simulink model "test_mdl1"  (R2023a)
settings: Solver=VariableStepAuto  StartTime=0.0  StopTime=10.0  RelTol=1e-3
(part 3 of 8)

== system test_mdl1/VehicleCAN/ECM_Diesel/Stop_Start ==
  AutoStopPtDelta_I_Est : Constant  Value=0
  HiElPwInhbt_B_Stat : Constant  Value=0
  OdoTripVerify_L_Actl : Constant  Value=0
  StopStrtDrvMde_D_Indic : Constant  Value=0
  StopStrtIODTxt_D_Rq : Constant  Value=0
  StopStrtMsgTxt_D_Rq : Constant  Value=0
  StopStrtStdby_D_Indic : Constant  Value=0
  bus_creator : BusCreator  Inputs=7
  out_port : Outport
  wires:
  bus_creator/1 -> out_port/1  "test_mdl1"
  AutoStopPtDelta_I_Est/1 -> bus_creator/1  "AutoStopPtDelta_I_Est"
  HiElPwInhbt_B_Stat/1 -> bus_creator/2  "HiElPwInhbt_B_Stat"
  OdoTripVerify_L_Actl/1 -> bus_creator/3  "OdoTripVerify_L_Actl"
  StopStrtDrvMde_D_Indic/1 -> bus_creator/4  "StopStrtDrvMde_D_Indic"
  StopStrtIODTxt_D_Rq/1 -> bus_creator/5  "StopStrtIODTxt_D_Rq"
  StopStrtMsgTxt_D_Rq/1 -> bus_creator/6  "StopStrtMsgTxt_D_Rq"
  StopStrtStdby_D_Indic/1 -> bus_creator/7  "StopStrtStdby_D_Indic"

== system test_mdl1/VehicleCAN/ECM_Diesel/TesterPhysicalResPCM ==
  TesterPhysicalResPCM : Constant  Value=0
  bus_creator : BusCreator  Inputs=1
  out_port : Outport
  wires:
  bus_creator/1 -> out_port/1  "test_mdl1"
  TesterPhysicalResPCM/1 -> bus_creator/1  "TesterPhysicalResPCM"

== system test_mdl1/VehicleCAN/ECM_Diesel/TesterPhysicalResSOBDMCFD1 ==
  TesterPhysicalResSOBDMC : Constant  Value=0
  bus_creator : BusCreator  Inputs=1
  out_port : Outport
  wires:
  bus_creator/1 -> out_port/1  "test_mdl1"
  TesterPhysicalResSOBDMC/1 -> bus_creator/1  "TesterPhysicalResSOBDMC"

== system test_mdl1/VehicleCAN/ECM_Diesel/TorqueDataEngFlags ==
  PrplWhlTotTqRq_No_Cnt : Constant  Value=0
  PrplWhlTotTqRq_No_Cs : Constant  Value=0
  PrplWhlTot_Tq_LimMn : Constant  Value=0
  PrplWhlTot_Tq_Rq : Constant  Value=0
  PtDrvMde_D_Stat : Constant  Value=0
  bus_creator : BusCreator  Inputs=5
  out_port : Outport
  wires:
  bus_creator/1 -> out_port/1  "test_mdl1"
  PrplWhlTotTqRq_No_Cnt/1 -> bus_creator/1  "PrplWhlTotTqRq_No_Cnt"
  PrplWhlTotTqRq_No_Cs/1 -> bus_creator/2  "PrplWhlTotTqRq_No_Cs"
  PrplWhlTot_Tq_LimMn/1 -> bus_creator/3  "PrplWhlTot_Tq_LimMn"
  PrplWhlTot_Tq_Rq/1 -> bus_creator/4  "PrplWhlTot_Tq_Rq"
  PtDrvMde_D_Stat/1 -> bus_creator/5  "PtDrvMde_D_Stat"

== system test_mdl1/VehicleCAN/ECM_Diesel/VehicleOperatingModes ==
  ElPw_D_Stat : Constant  Value=0
  ElPw_D_StatStrtStop : Constant  Value=0
  Eng_D_Stat : Constant  Value=0
  PlgActvArb_B_Actl : Constant  Value=0
  PrplWhlRgenMn_Tq_Actl : Constant  Value=0
  PrplWhlTot2_Tq_Actl : Constant  Value=0
  PwPckTq_D_Stat : Constant  Value=0
  TrnAinTq_D_Qf : Constant  Value=0
  TrnAin_Tq_Actl : Constant  Value=0
  bus_creator : BusCreator  Inputs=9
  out_port : Outport
  wires:
  bus_creator/1 -> out_port/1  "test_mdl1"
  ElPw_D_Stat/1 -> bus_creator/1  "ElPw_D_Stat"
  ElPw_D_StatStrtStop/1 -> bus_creator/2  "ElPw_D_StatStrtStop"
  Eng_D_Stat/1 -> bus_creator/3  "Eng_D_Stat"
  PlgActvArb_B_Actl/1 -> bus_creator/4  "PlgActvArb_B_Actl"
  PrplWhlRgenMn_Tq_Actl/1 -> bus_creator/5  "PrplWhlRgenMn_Tq_Actl"
  PrplWhlTot2_Tq_Actl/1 -> bus_creator/6  "PrplWhlTot2_Tq_Actl"
  PwPckTq_D_Stat/1 -> bus_creator/7  "PwPckTq_D_Stat"
  TrnAinTq_D_Qf/1 -> bus_creator/8  "TrnAinTq_D_Qf"
  TrnAin_Tq_Actl/1 -> bus_creator/9  "TrnAin_Tq_Actl"

== system test_mdl1/VehicleCAN/GWM/%sonality_APIM_Data_FD1 ==
  %s1OptIn_B_Stats : Constant  Value=0
  %s2OptIn_B_Stats : Constant  Value=0
  %s3OptIn_B_Stats : Constant  Value=0
  %s4OptIn_B_Stats : Constant  Value=0
  %sStore_D_Rq : Constant  Value=0
  CtrStk%sIndex_D_Actl : Constant  Value=0
  CtrStkDsplyOp_D_Rq : Constant  Value=0
  CtrStkFeatConfigActl : Constant  Value=0
  CtrStkFeatNoActl : Constant  Value=0
  bus_creator : BusCreator  Inputs=9
  out_port : Outport
  wires:
  bus_creator/1 -> out_port/1  "test_mdl1"
  CtrStkDsplyOp_D_Rq/1 -> bus_creator/1  "CtrStkDsplyOp_D_Rq"
  CtrStkFeatConfigActl/1 -> bus_creator/2  "CtrStkFeatConfigActl"
  CtrStkFeatNoActl/1 -> bus_creator/3  "CtrStkFeatNoActl"
  CtrStk%sIndex_D_Actl/1 -> bus_creator/4  "CtrStk%sIndex_D_Actl"
  %s1OptIn_B_Stats/1 -> bus_creator/5  "%s1OptIn_B_Stats"
  %s2OptIn_B_Stats/1 -> bus_creator/6  "%s2OptIn_B_Stats"
  %s3OptIn_B_Stats/1 -> bus_creator/7  "%s3OptIn_B_Stats"
  %s4OptIn_B_Stats/1 -> bus_creator/8  "%s4OptIn_B_Stats"
  %sStore_D_Rq/1 -> bus_creator/9  "%sStore_D_Rq"

== system test_mdl1/VehicleCAN/GWM/%sonality_BCM2_Data_FD1 ==
  %s1Key_D_Stat : Constant  Value=0
  %s2Key_D_Stat : Constant  Value=0
  %s3Key_D_Stat : Constant  Value=0
  %s4Key_D_Stat : Constant  Value=0
  %sConflict_D_Actl : Constant  Value=0
  %sNoPos_D_Actl : Constant  Value=0
  %sNo_D_Actl : Constant  Value=0
  %sRecallSrc_D_Actl : Constant  Value=0
  %sSetupAccessCtrl : Constant  Value=0
  %sSetupRestr_D_Actl : Constant  Value=0
  %sSetup_No_Actl : Constant  Value=0
  AssocConfirm_D_Actl : Constant  Value=0
  EmPrflKeyAssoc_D_Stat : Constant  Value=0
  EmPrflNo_D_Stat : Constant  Value=0
  RecallEvent_No_Cnt : Constant  Value=0
  VehKeyActv_D_Stat : Constant  Value=0
  bus_creator : BusCreator  Inputs=16
  out_port : Outport
  wires:
  bus_creator/1 -> out_port/1  "test_mdl1"
  AssocConfirm_D_Actl/1 -> bus_creator/1  "AssocConfirm_D_Actl"
  EmPrflKeyAssoc_D_Stat/1 -> bus_creator/2  "EmPrflKeyAssoc_D_Stat"
  EmPrflNo_D_Stat/1 -> bus_creator/3  "EmPrflNo_D_Stat"
  %s1Key_D_Stat/1 -> bus_creator/4  "%s1Key_D_Stat"
  %s2Key_D_Stat/1 -> bus_creator/5  "%s2Key_D_Stat"
  %s3Key_D_Stat/1 -> bus_creator/6  "%s3Key_D_Stat"
  %s4Key_D_Stat/1 -> bus_creator/7  "%s4Key_D_Stat"
  %sConflict_D_Actl/1 -> bus_creator/8  "%sConflict_D_Actl"
  %sNoPos_D_Actl/1 -> bus_creator/9  "%sNoPos_D_Actl"
  %sNo_D_Actl/1 -> bus_creator/10  "%sNo_D_Actl"
  %sRecallSrc_D_Actl/1 -> bus_creator/11  "%sRecallSrc_D_Actl"
  %sSetupAccessCtrl/1 -> bus_creator/12  "%sSetupAccessCtrl"
  %sSetupRestr_D_Actl/1 -> bus_creator/13  "%sSetupRestr_D_Actl"
  %sSetup_No_Actl/1 -> bus_creator/14  "%sSetup_No_Actl"
  RecallEvent_No_Cnt/1 -> bus_creator/15  "RecallEvent_No_Cnt"
  VehKeyActv_D_Stat/1 -> bus_creator/16  "VehKeyActv_D_Stat"

== system test_mdl1/VehicleCAN/GWM/%sonality_Data_FD1 ==
  MsgCntr%sIndex_D_Rq : Constant  Value=0
  MsgCntrDsplyOp_D_Rq : Constant  Value=0
  MsgCntrFeatConfigRq : Constant  Value=0
  MsgCntrFeatNoRq : Constant  Value=0
  bus_creator : BusCreator  Inputs=4
  out_port : Outport
  wires:
  bus_creator/1 -> out_port/1  "test_mdl1"
  MsgCntrDsplyOp_D_Rq/1 -> bus_creator/1  "MsgCntrDsplyOp_D_Rq"
  MsgCntrFeatConfigRq/1 -> bus_creator/2  "MsgCntrFeatConfigRq"
  MsgCntrFeatNoRq/1 -> bus_creator/3  "MsgCntrFeatNoRq"
  MsgCntr%sIndex_D_Rq/1 -> bus_creator/4  "MsgCntr%sIndex_D_Rq"

== system test_mdl1/VehicleCAN/GWM/AC_Compressor_Data_FD1 ==
  ElCmpr%fErr_D_Falt : Constant  Value=0
  ElCmprBattSysU_D_Falt : Constant  Value=0
  ElCmprBattURng_D_Falt : Constant  Value=0
  ElCmprInnrErr_D_Falt : Constant  Value=0
  ElCmprLostComm_D_Falt : Constant  Value=0
  ElCmprOverLoad_D_Falt : Constant  Value=0
  ElCmprOverTe_D_Falt : Constant  Value=0
  ElCmprOverTe_D_Stat : Constant  Value=0
  ElCmprSysU_D_Falt : Constant  Value=0
  ElCmprUHi_D_Stat : Constant  Value=0
  ElCmprUHi_U_Actl : Constant  Value=0
  ElCmpr_D_Stat : Constant  Value=0
  ElCmpr_N_Actl : Constant  Value=0
  ElCmpr_Pw_Actl : Constant  Value=0
  bus_creator : BusCreator  Inputs=14
  out_port : Outport
  wires:
  bus_creator/1 -> out_port/1  "test_mdl1"
  ElCmprBattSysU_D_Falt/1 -> bus_creator/1  "ElCmprBattSysU_D_Falt"
  ElCmprBattURng_D_Falt/1 -> bus_creator/2  "ElCmprBattURng_D_Falt"
  ElCmprInnrErr_D_Falt/1 -> bus_creator/3  "ElCmprInnrErr_D_Falt"
  ElCmprLostComm_D_Falt/1 -> bus_creator/4  "ElCmprLostComm_D_Falt"
  ElCmprOverLoad_D_Falt/1 -> bus_creator/5  "ElCmprOverLoad_D_Falt"
  ElCmprOverTe_D_Falt/1 -> bus_creator/6  "ElCmprOverTe_D_Falt"
  ElCmprOverTe_D_Stat/1 -> bus_creator/7  "ElCmprOverTe_D_Stat"
  ElCmpr%fErr_D_Falt/1 -> bus_creator/8  "ElCmpr%fErr_D_Falt"
  ElCmprSysU_D_Falt/1 -> bus_creator/9  "ElCmprSysU_D_Falt"
  ElCmprUHi_D_Stat/1 -> bus_creator/10  "ElCmprUHi_D_Stat"
  ElCmprUHi_U_Actl/1 -> bus_creator/11  "ElCmprUHi_U_Actl"
  ElCmpr_D_Stat/1 -> bus_creator/12  "ElCmpr_D_Stat"
  ElCmpr_N_Actl/1 -> bus_creator/13  "ElCmpr_N_Actl"
  ElCmpr_Pw_Actl/1 -> bus_creator/14  "ElCmpr_Pw_Actl"

== system test_mdl1/VehicleCAN/GWM/APIMGPS_Data_Nav_1_FD1 ==
  GPS_Latitude_Degrees : Constant  Value=0
  GPS_Latitude_Min_dec : Constant  Value=0
  GPS_Latitude_Minutes : Constant  Value=0
  GPS_Longitude_Degrees : Constant  Value=0
  GPS_Longitude_Min_dec : Constant  Value=0
  GPS_Longitude_Minutes : Constant  Value=0
  GpsHsphLattSth_D_Actl : Constant  Value=0
  GpsHsphLongEast_D_Actl : Constant  Value=0
  bus_creator : BusCreator  Inputs=8
  out_port : Outport
  wires:
  bus_creator/1 -> out_port/1  "test_mdl1"
  GPS_Latitude_Degrees/1 -> bus_creator/1  "GPS_Latitude_Degrees"
  GPS_Latitude_Min_dec/1 -> bus_creator/2  "GPS_Latitude_Min_dec"
  GPS_Latitude_Minutes/1 -> bus_creator/3  "GPS_Latitude_Minutes"
  GPS_Longitude_Degrees/1 -> bus_creator/4  "GPS_Longitude_Degrees"
  GPS_Longitude_Min_dec/1 -> bus_creator/5  "GPS_Longitude_Min_dec"
  GPS_Longitude_Minutes/1 -> bus_creator/6  "GPS_Longitude_Minutes"
  GpsHsphLattSth_D_Actl/1 -> bus_creator/7  "GpsHsphLattSth_D_Actl"
  GpsHsphLongEast_D_Actl/1 -> bus_creator/8  "GpsHsphLongEast_D_Actl"

== system test_mdl1/VehicleCAN/GWM/APIMGPS_Data_Nav_2_FD1 ==
  GPS_Actual_vs_Infer_pos : Constant  Value=0
  GPS_Compass_direction : Constant  Value=0
  GPS_Pdop : Constant  Value=0
  GPS_UTC_hours : Constant  Value=0
  GPS_UTC_minutes : Constant  Value=0
  GPS_UTC_seconds : Constant  Value=0
  GpsUtcDay_No_Actl : Constant  Value=0
  GpsUtcMnth_No_Actl : Constant  Value=0
  GpsUtcYr_No_Actl : Constant  Value=0
  Gps_B_Falt : Constant  Value=0
  bus_creator : BusCreator  Inputs=10
  out_port : Outport
  wires:
  bus_creator/1 -> out_port/1  "test_mdl1"
  GPS_Actual_vs_Infer_pos/1 -> bus_creator/1  "GPS_Actual_vs_Infer_pos"
  GPS_Compass_direction/1 -> bus_creator/2  "GPS_Compass_direction"
  GPS_Pdop/1 -> bus_creator/3  "GPS_Pdop"
  GPS_UTC_hours/1 -> bus_creator/4  "GPS_UTC_hours"
  GPS_UTC_minutes/1 -> bus_creator/5  "GPS_UTC_minutes"
  GPS_UTC_seconds/1 -> bus_creator/6  "GPS_UTC_seconds"
  GpsUtcDay_No_Actl/1 -> bus_creator/7  "GpsUtcDay_No_Actl"
  GpsUtcMnth_No_Actl/1 -> bus_creator/8  "GpsUtcMnth_No_Actl"
  GpsUtcYr_No_Actl/1 -> bus_creator/9  "GpsUtcYr_No_Actl"
  Gps_B_Falt/1 -> bus_creator/10  "Gps_B_Falt"

== system test_mdl1/VehicleCAN/GWM/APIMGPS_Data_Nav_3_FD1 ==
  GPS_Hdop : Constant  Value=0
  GPS_Heading : Constant  Value=0
  GPS_MSL_altitude : Constant  Value=0
  GPS_Sat_num_in_view : Constant  Value=0
  GPS_Speed : Constant  Value=0
  GPS_Vdop : Constant  Value=0
  GPS_dimension : Constant  Value=0
  bus_creator : BusCreator  Inputs=7
  out_port : Outport
  wires:
  bus_creator/1 -> out_port/1  "test_mdl1"
  GPS_Hdop/1 -> bus_creator/1  "GPS_Hdop"
  GPS_Heading/1 -> bus_creator/2  "GPS_Heading"
  GPS_MSL_altitude/1 -> bus_creator/3  "GPS_MSL_altitude"
  GPS_Sat_num_in_view/1 -> bus_creator/4  "GPS_Sat_num_in_view"
  GPS_Speed/1 -> bus_creator/5  "GPS_Speed"
  GPS_Vdop/1 -> bus_creator/6  "GPS_Vdop"
  GPS_dimension/1 -> bus_creator/7  "GPS_dimension"

== system test_mdl1/VehicleCAN/GWM/APIM_Data_FD1 ==
  AutoLghtOvrrd_B_RqDrv : Constant  Value=0
  DistToStopover_L_Actl : Constant  Value=0
  ExtLghtDsply_D_Stat : Constant  Value=0
  ExtLghtFront_D_RqMnu : Constant  Value=0
  ExtLghtLeft_D_RqMnu : Constant  Value=0
  ExtLghtRear_D_RqMnu : Constant  Value=0
  ExtLghtRight_D_RqMnu : Constant  Value=0
  GoTEditHr_T_RqMnu : Constant  Value=0
  GoTEditMnte_T_RqMnu : Constant  Value=0
  StopoverType_D_Stat : Constant  Value=0
  bus_creator : BusCreator  Inputs=10
  out_port : Outport
  wires:
  bus_creator/1 -> out_port/1  "test_mdl1"
  AutoLghtOvrrd_B_RqDrv/1 -> bus_creator/1  "AutoLghtOvrrd_B_RqDrv"
  DistToStopover_L_Actl/1 -> bus_creator/2  "DistToStopover_L_Actl"
  ExtLghtDsply_D_Stat/1 -> bus_creator/3  "ExtLghtDsply_D_Stat"
  ExtLghtFront_D_RqMnu/1 -> bus_creator/4  "ExtLghtFront_D_RqMnu"
  ExtLghtLeft_D_RqMnu/1 -> bus_creator/5  "ExtLghtLeft_D_RqMnu"
  ExtLghtRear_D_RqMnu/1 -> bus_creator/6  "ExtLghtRear_D_RqMnu"
  ExtLghtRight_D_RqMnu/1 -> bus_creator/7  "ExtLghtRight_D_RqMnu"
  GoTEditHr_T_RqMnu/1 -> bus_creator/8  "GoTEditHr_T_RqMnu"
  GoTEditMnte_T_RqMnu/1 -> bus_creator/9  "GoTEditMnte_T_RqMnu"
  StopoverType_D_Stat/1 -> bus_creator/10  "StopoverType_D_Stat"

== system test_mdl1/VehicleCAN/GWM/APIM_Request_Signals_1_FD1 ==
  Btt_L_Actl2 : Constant  Value=0
  ChrgCrdLckEnbl_B_Stat : Constant  Value=0
  ChrgOvrdExitScrn_D_Rq : Constant  Value=0
  Cntr_Plg_Mode_Cmd : Constant  Value=0
  EmPrflButtnAssoc_D_Rq : Constant  Value=0
  EmPrflKeyAssoc_D_Rq : Constant  Value=0
  EmPrflNo_D_Rq : Constant  Value=0
  Em_D_Stat : Constant  Value=0
  PmCabnLvl_D_Stat : Constant  Value=0
  PmCabn_D_Stat : Constant  Value=0
  PwRnngBoardMde_D_Rq : Constant  Value=0
  PwRnngBoardSwtch_D_Rq : Constant  Value=0
  PwRnngBoardT_D_Rq : Constant  Value=0
  Rba_D_Rq : Constant  Value=0
  bus_creator : BusCreator  Inputs=14
  out_port : Outport
  wires:
  bus_creator/1 -> out_port/1  "test_mdl1"
  Btt_L_Actl2/1 -> bus_creator/1  "Btt_L_Actl2"
  ChrgCrdLckEnbl_B_Stat/1 -> bus_creator/2  "ChrgCrdLckEnbl_B_Stat"
  ChrgOvrdExitScrn_D_Rq/1 -> bus_creator/3  "ChrgOvrdExitScrn_D_Rq"
  Cntr_Plg_Mode_Cmd/1 -> bus_creator/4  "Cntr_Plg_Mode_Cmd"
  EmPrflButtnAssoc_D_Rq/1 -> bus_creator/5  "EmPrflButtnAssoc_D_Rq"
  EmPrflKeyAssoc_D_Rq/1 -> bus_creator/6  "EmPrflKeyAssoc_D_Rq"
  EmPrflNo_D_Rq/1 -> bus_creator/7  "EmPrflNo_D_Rq"
  Em_D_Stat/1 -> bus_creator/8  "Em_D_Stat"
  PmCabnLvl_D_Stat/1 -> bus_creator/9  "PmCabnLvl_D_Stat"
  PmCabn_D_Stat/1 -> bus_creator/10  "PmCabn_D_Stat"
  PwRnngBoardMde_D_Rq/1 -> bus_creator/11  "PwRnngBoardMde_D_Rq"
  PwRnngBoardSwtch_D_Rq/1 -> bus_creator/12  "PwRnngBoardSwtch_D_Rq"
  PwRnngBoardT_D_Rq/1 -> bus_creator/13  "PwRnngBoardT_D_Rq"
  Rba_D_Rq/1 -> bus_creator/14  "Rba_D_Rq"

== system test_mdl1/VehicleCAN/GWM/APIM_Request_Signals_5_FD1 ==
  OnbChrgLocIdTrgt_No_Rq : Constant  Value=0
  OnbChrgLocIdUns_B_Rq : Constant  Value=0
  OnbChrgPrflUpdate_B_Rq : Constant  Value=0
  OnbChrgPrflWkdy_No_Rq : Constant  Value=0
  OnbChrgPrflWknd_No_Rq : Constant  Value=0
  OnbChrgSetDelete_B_Rq : Constant  Value=0
  OnbChrgSetNow_D_Rq : Constant  Value=0
  OnbChrgToPcWkdy_D_Actl : Constant  Value=0
  OnbChrgToPcWknd_D_Actl : Constant  Value=0
  bus_creator : BusCreator  Inputs=9
  out_port : Outport
  wires:
  bus_creator/1 -> out_port/1  "test_mdl1"
  OnbChrgLocIdTrgt_No_Rq/1 -> bus_creator/1  "OnbChrgLocIdTrgt_No_Rq"
  OnbChrgLocIdUns_B_Rq/1 -> bus_creator/2  "OnbChrgLocIdUns_B_Rq"
  OnbChrgPrflUpdate_B_Rq/1 -> bus_creator/3  "OnbChrgPrflUpdate_B_Rq"
  OnbChrgPrflWkdy_No_Rq/1 -> bus_creator/4  "OnbChrgPrflWkdy_No_Rq"
  OnbChrgPrflWknd_No_Rq/1 -> bus_creator/5  "OnbChrgPrflWknd_No_Rq"
  OnbChrgSetDelete_B_Rq/1 -> bus_creator/6  "OnbChrgSetDelete_B_Rq"
  OnbChrgSetNow_D_Rq/1 -> bus_creator/7  "OnbChrgSetNow_D_Rq"
  OnbChrgToPcWkdy_D_Actl/1 -> bus_creator/8  "OnbChrgToPcWkdy_D_Actl"
  OnbChrgToPcWknd_D_Actl/1 -> bus_creator/9  "OnbChrgToPcWknd_D_Actl"

== system test_mdl1/VehicleCAN/GWM/APIM_Request_Signals_FD1 ==
  CbnCmrtPrefListIndx_Rq : Constant  Value=0
  CbnCmrtPrefLstNmItm_Rq : Constant  Value=0
  ChrgStatDsply_D_Rq : Constant  Value=0
  FactoryReset_Rq : Constant  Value=0
  LongTermParking_Rq : Constant  Value=0
  ModemReset_D_Rq : Constant  Value=0
  NextUsageTimeToggle_Rq : Constant  Value=0
  OffPeakTimeSetHR_Rq : Constant  Value=0
  OffPeakTimeSetMin_Rq : Constant  Value=0
  StopStrtDrvMde_B_RqBtn3 : Constant  Value=0
  TCU_ESN_D_Rq : Constant  Value=0
  bus_creator : BusCreator  Inputs=11
  out_port : Outport
  wires:
  bus_creator/1 -> out_port/1  "test_mdl1"
  CbnCmrtPrefListIndx_Rq/1 -> bus_creator/1  "CbnCmrtPrefListIndx_Rq"
  CbnCmrtPrefLstNmItm_Rq/1 -> bus_creator/2  "CbnCmrtPrefLstNmItm_Rq"
  ChrgStatDsply_D_Rq/1 -> bus_creator/3  "ChrgStatDsply_D_Rq"
  FactoryReset_Rq/1 -> bus_creator/4  "FactoryReset_Rq"
  LongTermParking_Rq/1 -> bus_creator/5  "LongTermParking_Rq"
  ModemReset_D_Rq/1 -> bus_creator/6  "ModemReset_D_Rq"
  NextUsageTimeToggle_Rq/1 -> bus_creator/7  "NextUsageTimeToggle_Rq"
  OffPeakTimeSetHR_Rq/1 -> bus_creator/8  "OffPeakTimeSetHR_Rq"
  OffPeakTimeSetMin_Rq/1 -> bus_creator/9  "OffPeakTimeSetMin_Rq"
  StopStrtDrvMde_B_RqBtn3/1 -> bus_creator/10  "StopStrtDrvMde_B_RqBtn3"
  TCU_ESN_D_Rq/1 -> bus_creator/11  "TCU_ESN_D_Rq"

== system test_mdl1/VehicleCAN/GWM/APIM_Send_Signals1_FD1 ==
  APIM_ActiveTrackNum_St : Constant  Value=0
  APIM_NumberofTracks_St : Constant  Value=0
  AutoHoldSwtch_D_Stat3 : Constant  Value=0
  CenterStackRing_D_Actl : Constant  Value=0
  ChrgCordUnlock_B_Rq : Constant  Value=0
  TrlrAidCancl_B_Rq : Constant  Value=0
  TrlrAidSetup_D_Stat : Constant  Value=0
  TrlrTrgtAcquire_D_Rq : Constant  Value=0
  ValetMode_D_Stat : Constant  Value=0
  bus_creator : BusCreator  Inputs=9
  out_port : Outport
  wires:
  bus_creator/1 -> out_port/1  "test_mdl1"
  APIM_ActiveTrackNum_St/1 -> bus_creator/1  "APIM_ActiveTrackNum_St"
  APIM_NumberofTracks_St/1 -> bus_creator/2  "APIM_NumberofTracks_St"
  AutoHoldSwtch_D_Stat3/1 -> bus_creator/3  "AutoHoldSwtch_D_Stat3"
  CenterStackRing_D_Actl/1 -> bus_creator/4  "CenterStackRing_D_Actl"
  ChrgCordUnlock_B_Rq/1 -> bus_creator/5  "ChrgCordUnlock_B_Rq"
  TrlrAidCancl_B_Rq/1 -> bus_creator/6  "TrlrAidCancl_B_Rq"
  TrlrAidSetup_D_Stat/1 -> bus_creator/7  "TrlrAidSetup_D_Stat"
  TrlrTrgtAcquire_D_Rq/1 -> bus_creator/8  "TrlrTrgtAcquire_D_Rq"
  ValetMode_D_Stat/1 -> bus_creator/9  "ValetMode_D_Stat"

== system test_mdl1/VehicleCAN/GWM/APIM_Send_Signals_2_FD1 ==
  AutoEpbButtn_B_Stat : Constant  Value=0
  AutoEpbZoomView_B_Stat : Constant  Value=0
  DcacGfciTestBttn_B_Stat : Constant  Value=0
  DcacPwButtn_B_Falt : Constant  Value=0
  DcacPwHiButtn_B_Stat : Constant  Value=0
  DcacPwLoButtn_B_Stat : Constant  Value=0
  DcacPwOffButtn_B_Stat : Constant  Value=0
  DcacPwResetButtn_B_Stat : Constant  Value=0
  OnbChrgClearAll_B_Rq : Constant  Value=0
  OnbChrgGoTDelete_B_Rq : Constant  Value=0
  OnbChrgGoTElement_D_Rq : Constant  Value=0
  OnbChrgGoTExtHtr_D_Rq : Constant  Value=0
  OnbChrgGoTHr_T_Rq : Constant  Value=0
  OnbChrgGoTMnte_D_Rq : Constant  Value=0
  OnbChrgGoTOn_D_Rq : Constant  Value=0
  OnbChrgGoTPrcond_D_Rq : Constant  Value=0
  OnbChrgGoTTouch_D_Rq : Constant  Value=0
  OnbChrgGoTUpdate_B_Rq : Constant  Value=0
  OtaTrg_D_Stat : Constant  Value=0
  PaakMyKey_D_Rq : Constant  Value=0
  TCU_Final_Actvtn_St : Constant  Value=0
  TCU_Init_Actvtn_St : Constant  Value=0
  TrlrAidMde_D_Rq : Constant  Value=0
  TrlrBrkGain_No_Rq : Constant  Value=0
  TrlrHitch_D_RqMnu : Constant  Value=0
  bus_creator : BusCreator  Inputs=25
  out_port : Outport
  wires:
  bus_creator/1 -> out_port/1  "test_mdl1"
  AutoEpbButtn_B_Stat/1 -> bus_creator/1  "AutoEpbButtn_B_Stat"
  AutoEpbZoomView_B_Stat/1 -> bus_creator/2  "AutoEpbZoomView_B_Stat"
  DcacGfciTestBttn_B_Stat/1 -> bus_creator/3  "DcacGfciTestBttn_B_Stat"
  DcacPwButtn_B_Falt/1 -> bus_creator/4  "DcacPwButtn_B_Falt"
  DcacPwHiButtn_B_Stat/1 -> bus_creator/5  "DcacPwHiButtn_B_Stat"
  DcacPwLoButtn_B_Stat/1 -> bus_creator/6  "DcacPwLoButtn_B_Stat"
  DcacPwOffButtn_B_Stat/1 -> bus_creator/7  "DcacPwOffButtn_B_Stat"
  DcacPwResetButtn_B_Stat/1 -> bus_creator/8  "DcacPwResetButtn_B_Stat"
  OnbChrgClearAll_B_Rq/1 -> bus_creator/9  "OnbChrgClearAll_B_Rq"
  OnbChrgGoTDelete_B_Rq/1 -> bus_creator/10  "OnbChrgGoTDelete_B_Rq"
  OnbChrgGoTElement_D_Rq/1 -> bus_creator/11  "OnbChrgGoTElement_D_Rq"
  OnbChrgGoTExtHtr_D_Rq/1 -> bus_creator/12  "OnbChrgGoTExtHtr_D_Rq"
  OnbChrgGoTHr_T_Rq/1 -> bus_creator/13  "OnbChrgGoTHr_T_Rq"
  OnbChrgGoTMnte_D_Rq/1 -> bus_creator/14  "OnbChrgGoTMnte_D_Rq"
  OnbChrgGoTOn_D_Rq/1 -> bus_creator/15  "OnbChrgGoTOn_D_Rq"
  OnbChrgGoTPrcond_D_Rq/1 -> bus_creator/16  "OnbChrgGoTPrcond_D_Rq"
  OnbChrgGoTTouch_D_Rq/1 -> bus_creator/17  "OnbChrgGoTTouch_D_Rq"
  OnbChrgGoTUpdate_B_Rq/1 -> bus_creator/18  "OnbChrgGoTUpdate_B_Rq"
  OtaTrg_D_Stat/1 -> bus_creator/19  "OtaTrg_D_Stat"
  PaakMyKey_D_Rq/1 -> bus_creator/20  "PaakMyKey_D_Rq"
  TCU_Final_Actvtn_St/1 -> bus_creator/21  "TCU_Final_Actvtn_St"
  TCU_Init_Actvtn_St/1 -> bus_creator/22  "TCU_Init_Actvtn_St"
  TrlrAidMde_D_Rq/1 -> bus_creator/23  "TrlrAidMde_D_Rq"
  TrlrBrkGain_No_Rq/1 -> bus_creator/24  "TrlrBrkGain_No_Rq"
  TrlrHitch_D_RqMnu/1 -> bus_creator/25  "TrlrHitch_D_RqMnu"

== system test_mdl1/VehicleCAN/GWM/Accel_Data_FD1 ==
  VehLat2_A_Actl : Constant  Value=0
  VehLatAActl_D_Qf : Constant  Value=0
  VehLatLongVertA_No_Cs : Constant  Value=0
  VehLatLongVert_No_Cnt : Constant  Value=0
  VehLong2_A_Actl : Constant  Value=0
  VehLongAActl_D_Qf : Constant  Value=0
  VehVert2_A_Actl : Constant  Value=0
  VehVertAActl_D_Qf : Constant  Value=0
  bus_creator : BusCreator  Inputs=8
  out_port : Outport
  wires:
  bus_creator/1 -> out_port/1  "test_mdl1"
  VehLat2_A_Actl/1 -> bus_creator/1  "VehLat2_A_Actl"
  VehLatAActl_D_Qf/1 -> bus_creator/2  "VehLatAActl_D_Qf"
  VehLatLongVertA_No_Cs/1 -> bus_creator/3  "VehLatLongVertA_No_Cs"
  VehLatLongVert_No_Cnt/1 -> bus_creator/4  "VehLatLongVert_No_Cnt"
  VehLong2_A_Actl/1 -> bus_creator/5  "VehLong2_A_Actl"
  VehLongAActl_D_Qf/1 -> bus_creator/6  "VehLongAActl_D_Qf"
  VehVert2_A_Actl/1 -> bus_creator/7  "VehVert2_A_Actl"
  VehVertAActl_D_Qf/1 -> bus_creator/8  "VehVertAActl_D_Qf"

== system test_mdl1/VehicleCAN/GWM/ActiveFrontStrg_Stat2_FD1 ==
  SteWhlRelCalib_An_Sns : Constant  Value=0
  SteWhlRelCalib_T_Actl : Constant  Value=0
  bus_creator : BusCreator  Inputs=2
  out_port : Outport
  wires:
  bus_creator/1 -> out_port/1  "test_mdl1"
  SteWhlRelCalib_An_Sns/1 -> bus_creator/1  "SteWhlRelCalib_An_Sns"
  SteWhlRelCalib_T_Actl/1 -> bus_creator/2  "SteWhlRelCalib_T_Actl"

== system test_mdl1/VehicleCAN/GWM/ActiveFrontStrg_Stat_FD1 ==
  SteWhlBrkAnActl_No_Cnt : Constant  Value=0
  SteWhlBrkAnActl_No_Cs : Constant  Value=0
  SteWhlBrkOffst_An_Actl : Constant  Value=0
  SteWhlOffstRq_D_Stat : Constant  Value=0
  SteWhlOffst_An_TotActl : Constant  Value=0
  bus_creator : BusCreator  Inputs=5
  out_port : Outport
  wires:
  bus_creator/1 -> out_port/1  "test_mdl1"
  SteWhlBrkAnActl_No_Cnt/1 -> bus_creator/1  "SteWhlBrkAnActl_No_Cnt"
  SteWhlBrkAnActl_No_Cs/1 -> bus_creator/2  "SteWhlBrkAnActl_No_Cs"
  SteWhlBrkOffst_An_Actl/1 -> bus_creator/3  "SteWhlBrkOffst_An_Actl"
  SteWhlOffstRq_D_Stat/1 -> bus_creator/4  "SteWhlOffstRq_D_Stat"
  SteWhlOffst_An_TotActl/1 -> bus_creator/5  "SteWhlOffst_An_TotActl"

== system test_mdl1/VehicleCAN/GWM/Adaptive_Headlamp_Stat ==
  Adaptive_Hdlmp_Fault : Constant  Value=0
  AhbStatGfhbFdbk_D_Actl : Constant  Value=0
  HeadLghtDrvSide_B_Stat : Constant  Value=0
  HeadLghtHiOn_B_StatHcm : Constant  Value=0
  bus_creator : BusCreator  Inputs=4
  out_port : Outport
  wires:
  bus_creator/1 -> out_port/1  "test_mdl1"
  Adaptive_Hdlmp_Fault/1 -> bus_creator/1  "Adaptive_Hdlmp_Fault"
  AhbStatGfhbFdbk_D_Actl/1 -> bus_creator/2  "AhbStatGfhbFdbk_D_Actl"
  HeadLghtDrvSide_B_Stat/1 -> bus_creator/3  "HeadLghtDrvSide_B_Stat"
  HeadLghtHiOn_B_StatHcm/1 -> bus_creator/4  "HeadLghtHiOn_B_StatHcm"

== system test_mdl1/VehicleCAN/GWM/AllTerrainControlData_FD1 ==
  SelDrvMdeCnt_D_Stat : Constant  Value=0
  SelDrvMdeSwtch_D_Stat : Constant  Value=0
  SelDrvMdeSwtch_No_Actl : Constant  Value=0
  bus_creator : BusCreator  Inputs=3
  out_port : Outport
  wires:
  bus_creator/1 -> out_port/1  "test_mdl1"
  SelDrvMdeCnt_D_Stat/1 -> bus_creator/1  "SelDrvMdeCnt_D_Stat"
  SelDrvMdeSwtch_D_Stat/1 -> bus_creator/2  "SelDrvMdeSwtch_D_Stat"
  SelDrvMdeSwtch_No_Actl/1 -> bus_creator/3  "SelDrvMdeSwtch_No_Actl"

== system test_mdl1/VehicleCAN/GWM/All_Terrain_Data_FD1 ==
  TerrMde_D_RqDrv : Constant  Value=0
  bus_creator : BusCreator  Inputs=1
  out_port : Outport
  wires:
  bus_creator/1 -> out_port/1  "test_mdl1"
  TerrMde_D_RqDrv/1 -> bus_creator/1  "TerrMde_D_RqDrv"

== system test_mdl1/VehicleCAN/GWM/BCMC_Data_FD1 ==
  WndwRearHeat_D_Stat : Constant  Value=0
  WndwRearHeat_I_Actl : Constant  Value=0
  bus_creator : BusCreator  Inputs=2
  out_port : Outport
  wires:
  bus_creator/1 -> out_port/1  "test_mdl1"
  WndwRearHeat_D_Stat/1 -> bus_creator/1  "WndwRearHeat_D_Stat"
  WndwRearHeat_I_Actl/1 -> bus_creator/2  "WndwRearHeat_I_Actl"

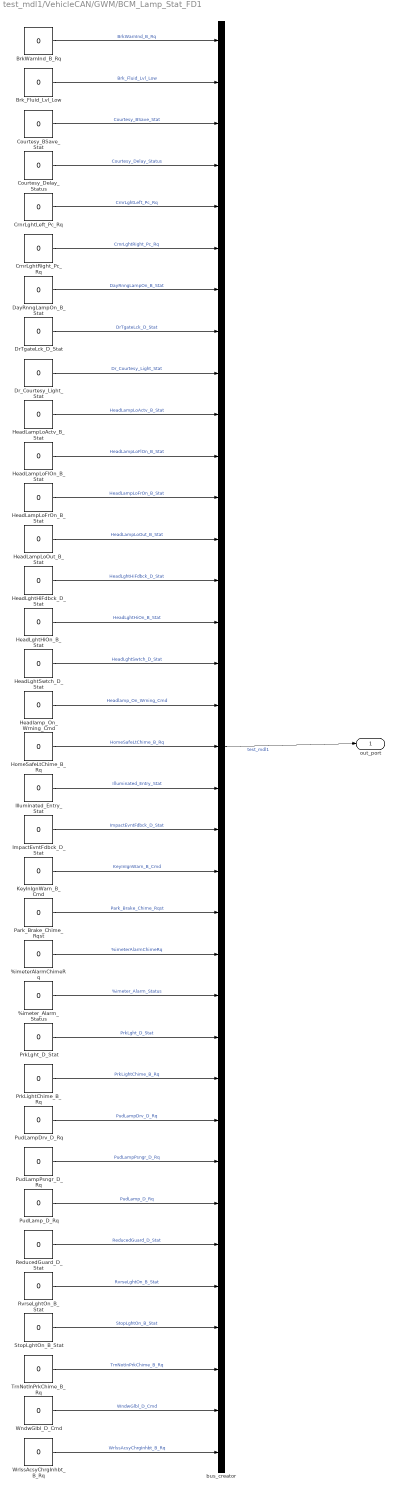
== system test_mdl1/VehicleCAN/GWM/BCM_Lamp_Stat_FD1 ==
  %imeterAlarmChimeRq : Constant  Value=0
  %imeter_Alarm_Status : Constant  Value=0
  BrkWarnInd_B_Rq : Constant  Value=0
  Brk_Fluid_Lvl_Low : Constant  Value=0
  Courtesy_BSave_Stat : Constant  Value=0
  Courtesy_Delay_Status : Constant  Value=0
  CrnrLghtLeft_Pc_Rq : Constant  Value=0
  CrnrLghtRight_Pc_Rq : Constant  Value=0
  DayRnngLampOn_B_Stat : Constant  Value=0
  DrTgateLck_D_Stat : Constant  Value=0
  Dr_Courtesy_Light_Stat : Constant  Value=0
  HeadLampLoActv_B_Stat : Constant  Value=0
  HeadLampLoFlOn_B_Stat : Constant  Value=0
  HeadLampLoFrOn_B_Stat : Constant  Value=0
  HeadLampLoOut_B_Stat : Constant  Value=0
  HeadLghtHiFdbck_D_Stat : Constant  Value=0
  HeadLghtHiOn_B_Stat : Constant  Value=0
  HeadLghtSwtch_D_Stat : Constant  Value=0
  Headlamp_On_Wrning_Cmd : Constant  Value=0
  HomeSafeLtChime_B_Rq : Constant  Value=0
  Illuminated_Entry_Stat : Constant  Value=0
  ImpactEvntFdbck_D_Stat : Constant  Value=0
  KeyInIgnWarn_B_Cmd : Constant  Value=0
  Park_Brake_Chime_Rqst : Constant  Value=0
  PrkLght_D_Stat : Constant  Value=0
  PrkLightChime_B_Rq : Constant  Value=0
  PudLampDrv_D_Rq : Constant  Value=0
  PudLampPsngr_D_Rq : Constant  Value=0
  PudLamp_D_Rq : Constant  Value=0
  ReducedGuard_D_Stat : Constant  Value=0
  RvrseLghtOn_B_Stat : Constant  Value=0
  StopLghtOn_B_Stat : Constant  Value=0
  TrnNotInPrkChime_B_Rq : Constant  Value=0
  WndwGlbl_D_Cmd : Constant  Value=0
  WrlssAcsyChrgInhbt_B_Rq : Constant  Value=0
  bus_creator : BusCreator  Inputs=35
  out_port : Outport
  wires:
  bus_creator/1 -> out_port/1  "test_mdl1"
  BrkWarnInd_B_Rq/1 -> bus_creator/1  "BrkWarnInd_B_Rq"
  Brk_Fluid_Lvl_Low/1 -> bus_creator/2  "Brk_Fluid_Lvl_Low"
  Courtesy_BSave_Stat/1 -> bus_creator/3  "Courtesy_BSave_Stat"
  Courtesy_Delay_Status/1 -> bus_creator/4  "Courtesy_Delay_Status"
  CrnrLghtLeft_Pc_Rq/1 -> bus_creator/5  "CrnrLghtLeft_Pc_Rq"
  CrnrLghtRight_Pc_Rq/1 -> bus_creator/6  "CrnrLghtRight_Pc_Rq"
  DayRnngLampOn_B_Stat/1 -> bus_creator/7  "DayRnngLampOn_B_Stat"
  DrTgateLck_D_Stat/1 -> bus_creator/8  "DrTgateLck_D_Stat"
  Dr_Courtesy_Light_Stat/1 -> bus_creator/9  "Dr_Courtesy_Light_Stat"
  HeadLampLoActv_B_Stat/1 -> bus_creator/10  "HeadLampLoActv_B_Stat"
  HeadLampLoFlOn_B_Stat/1 -> bus_creator/11  "HeadLampLoFlOn_B_Stat"
  HeadLampLoFrOn_B_Stat/1 -> bus_creator/12  "HeadLampLoFrOn_B_Stat"
  HeadLampLoOut_B_Stat/1 -> bus_creator/13  "HeadLampLoOut_B_Stat"
  HeadLghtHiFdbck_D_Stat/1 -> bus_creator/14  "HeadLghtHiFdbck_D_Stat"
  HeadLghtHiOn_B_Stat/1 -> bus_creator/15  "HeadLghtHiOn_B_Stat"
  HeadLghtSwtch_D_Stat/1 -> bus_creator/16  "HeadLghtSwtch_D_Stat"
  Headlamp_On_Wrning_Cmd/1 -> bus_creator/17  "Headlamp_On_Wrning_Cmd"
  HomeSafeLtChime_B_Rq/1 -> bus_creator/18  "HomeSafeLtChime_B_Rq"
  Illuminated_Entry_Stat/1 -> bus_creator/19  "Illuminated_Entry_Stat"
  ImpactEvntFdbck_D_Stat/1 -> bus_creator/20  "ImpactEvntFdbck_D_Stat"
  KeyInIgnWarn_B_Cmd/1 -> bus_creator/21  "KeyInIgnWarn_B_Cmd"
  Park_Brake_Chime_Rqst/1 -> bus_creator/22  "Park_Brake_Chime_Rqst"
  %imeterAlarmChimeRq/1 -> bus_creator/23  "%imeterAlarmChimeRq"
  %imeter_Alarm_Status/1 -> bus_creator/24  "%imeter_Alarm_Status"
  PrkLght_D_Stat/1 -> bus_creator/25  "PrkLght_D_Stat"
  PrkLightChime_B_Rq/1 -> bus_creator/26  "PrkLightChime_B_Rq"
  PudLampDrv_D_Rq/1 -> bus_creator/27  "PudLampDrv_D_Rq"
  PudLampPsngr_D_Rq/1 -> bus_creator/28  "PudLampPsngr_D_Rq"
  PudLamp_D_Rq/1 -> bus_creator/29  "PudLamp_D_Rq"
  ReducedGuard_D_Stat/1 -> bus_creator/30  "ReducedGuard_D_Stat"
  RvrseLghtOn_B_Stat/1 -> bus_creator/31  "RvrseLghtOn_B_Stat"
  StopLghtOn_B_Stat/1 -> bus_creator/32  "StopLghtOn_B_Stat"
  TrnNotInPrkChime_B_Rq/1 -> bus_creator/33  "TrnNotInPrkChime_B_Rq"
  WndwGlbl_D_Cmd/1 -> bus_creator/34  "WndwGlbl_D_Cmd"
  WrlssAcsyChrgInhbt_B_Rq/1 -> bus_creator/35  "WrlssAcsyChrgInhbt_B_Rq"

== system test_mdl1/VehicleCAN/GWM/BattRgenLo_1_FD1 ==
  BattRgenLo_I_Actl : Constant  Value=0
  BattRgenLo_U_Actl : Constant  Value=0
  bus_creator : BusCreator  Inputs=2
  out_port : Outport
  wires:
  bus_creator/1 -> out_port/1  "test_mdl1"
  BattRgenLo_I_Actl/1 -> bus_creator/1  "BattRgenLo_I_Actl"
  BattRgenLo_U_Actl/1 -> bus_creator/2  "BattRgenLo_U_Actl"

== system test_mdl1/VehicleCAN/GWM/BattRgenLo_2_FD1 ==
  BattRgenLoChrg_I_Mx : Constant  Value=0
  BattRgenLoChrg_U_Mx : Constant  Value=0
  BattRgenLoDchrg_I_Mx : Constant  Value=0
  BattRgenLoDchrg_U_Mn : Constant  Value=0
  BattRgenLoOpen_U_Actl : Constant  Value=0
  bus_creator : BusCreator  Inputs=5
  out_port : Outport
  wires:
  bus_creator/1 -> out_port/1  "test_mdl1"
  BattRgenLoChrg_I_Mx/1 -> bus_creator/1  "BattRgenLoChrg_I_Mx"
  BattRgenLoChrg_U_Mx/1 -> bus_creator/2  "BattRgenLoChrg_U_Mx"
  BattRgenLoDchrg_I_Mx/1 -> bus_creator/3  "BattRgenLoDchrg_I_Mx"
  BattRgenLoDchrg_U_Mn/1 -> bus_creator/4  "BattRgenLoDchrg_U_Mn"
  BattRgenLoOpen_U_Actl/1 -> bus_creator/5  "BattRgenLoOpen_U_Actl"

== system test_mdl1/VehicleCAN/GWM/BattRgenLo_3_FD1 ==
  BattRgenLoBalnc_B_Rq : Constant  Value=0
  BattRgenLo_AhRide_Actl : Constant  Value=0
  BattRgenLo_Ah_Actl : Constant  Value=0
  BattRgenLo_R_Actl : Constant  Value=0
  BattRgenLo_Te_Actl : Constant  Value=0
  BattRgenLo_Te_Hi : Constant  Value=0
  bus_creator : BusCreator  Inputs=6
  out_port : Outport
  wires:
  bus_creator/1 -> out_port/1  "test_mdl1"
  BattRgenLoBalnc_B_Rq/1 -> bus_creator/1  "BattRgenLoBalnc_B_Rq"
  BattRgenLo_AhRide_Actl/1 -> bus_creator/2  "BattRgenLo_AhRide_Actl"
  BattRgenLo_Ah_Actl/1 -> bus_creator/3  "BattRgenLo_Ah_Actl"
  BattRgenLo_R_Actl/1 -> bus_creator/4  "BattRgenLo_R_Actl"
  BattRgenLo_Te_Actl/1 -> bus_creator/5  "BattRgenLo_Te_Actl"
  BattRgenLo_Te_Hi/1 -> bus_creator/6  "BattRgenLo_Te_Hi"

== system test_mdl1/VehicleCAN/GWM/BattRgenLo_4_FD1 ==
  BattRgenLoChrg_B_Rq : Constant  Value=0
  BattRgenLoChrg_D_Stat : Constant  Value=0
  BattRgenLoDChrg_D_Stat : Constant  Value=0
  BattRgenLoDchrg_B_Rq : Constant  Value=0
  BattRgenLoPrtct_B_Stat : Constant  Value=0
  BattRgenLoPulse_U_Pred : Constant  Value=0
  BattRgenLoSoc_Pc_Actl : Constant  Value=0
  BattRgenLoStat_D_Qlty : Constant  Value=0
  BattRgenLo_B_Falt : Constant  Value=0
  BattRgenLo_T_Est : Constant  Value=0
  bus_creator : BusCreator  Inputs=10
  out_port : Outport
  wires:
  bus_creator/1 -> out_port/1  "test_mdl1"
  BattRgenLoChrg_B_Rq/1 -> bus_creator/1  "BattRgenLoChrg_B_Rq"
  BattRgenLoChrg_D_Stat/1 -> bus_creator/2  "BattRgenLoChrg_D_Stat"
  BattRgenLoDChrg_D_Stat/1 -> bus_creator/3  "BattRgenLoDChrg_D_Stat"
  BattRgenLoDchrg_B_Rq/1 -> bus_creator/4  "BattRgenLoDchrg_B_Rq"
  BattRgenLoPrtct_B_Stat/1 -> bus_creator/5  "BattRgenLoPrtct_B_Stat"
  BattRgenLoPulse_U_Pred/1 -> bus_creator/6  "BattRgenLoPulse_U_Pred"
  BattRgenLoSoc_Pc_Actl/1 -> bus_creator/7  "BattRgenLoSoc_Pc_Actl"
  BattRgenLoStat_D_Qlty/1 -> bus_creator/8  "BattRgenLoStat_D_Qlty"
  BattRgenLo_B_Falt/1 -> bus_creator/9  "BattRgenLo_B_Falt"
  BattRgenLo_T_Est/1 -> bus_creator/10  "BattRgenLo_T_Est"

== system test_mdl1/VehicleCAN/GWM/Battery_Mgmt_24V_FD1 ==
  BattULo24Soc_Pc_Actl : Constant  Value=0
  BattULo24State_D_Qlty : Constant  Value=0
  BattULo24_Ah_DeltaRide : Constant  Value=0
  BattULo24_B_Falt : Constant  Value=0
  BattULo24_D_Falt : Constant  Value=0
  BattULo24_I_Actl : Constant  Value=0
  BattULo24_Te_Actl : Constant  Value=0
  bus_creator : BusCreator  Inputs=7
  out_port : Outport
  wires:
  bus_creator/1 -> out_port/1  "test_mdl1"
  BattULo24Soc_Pc_Actl/1 -> bus_creator/1  "BattULo24Soc_Pc_Actl"
  BattULo24State_D_Qlty/1 -> bus_creator/2  "BattULo24State_D_Qlty"
  BattULo24_Ah_DeltaRide/1 -> bus_creator/3  "BattULo24_Ah_DeltaRide"
  BattULo24_B_Falt/1 -> bus_creator/4  "BattULo24_B_Falt"
  BattULo24_D_Falt/1 -> bus_creator/5  "BattULo24_D_Falt"
  BattULo24_I_Actl/1 -> bus_creator/6  "BattULo24_I_Actl"
  BattULo24_Te_Actl/1 -> bus_creator/7  "BattULo24_Te_Actl"

== system test_mdl1/VehicleCAN/GWM/Battery_Mgmt_2_FD1 ==
  %iodicElLoad_B_Stat : Constant  Value=0
  BattULoChrg_D_Rq : Constant  Value=0
  BattULoSrvc_T_Actl : Constant  Value=0
  Batt_Crit_SoC_B : Constant  Value=0
  Batt_Lo_SoC_B : Constant  Value=0
  ChargeMode : Constant  Value=0
  EngStrtInhbt_B_RqBatt : Constant  Value=0
  IdleSpeedIncrease_El : Constant  Value=0
  PwSysULoFalt_D_Stat : Constant  Value=0
  Shed_Drain_Eng_Off_B : Constant  Value=0
  Shed_Feature_Group_ID : Constant  Value=0
  Shed_Level_Req : Constant  Value=0
  Shed_T_Eng_Off_B : Constant  Value=0
  ULoRgenTestMde_B_Rq : Constant  Value=0
  bus_creator : BusCreator  Inputs=14
  out_port : Outport
  wires:
  bus_creator/1 -> out_port/1  "test_mdl1"
  BattULoChrg_D_Rq/1 -> bus_creator/1  "BattULoChrg_D_Rq"
  BattULoSrvc_T_Actl/1 -> bus_creator/2  "BattULoSrvc_T_Actl"
  Batt_Crit_SoC_B/1 -> bus_creator/3  "Batt_Crit_SoC_B"
  Batt_Lo_SoC_B/1 -> bus_creator/4  "Batt_Lo_SoC_B"
  ChargeMode/1 -> bus_creator/5  "ChargeMode"
  EngStrtInhbt_B_RqBatt/1 -> bus_creator/6  "EngStrtInhbt_B_RqBatt"
  IdleSpeedIncrease_El/1 -> bus_creator/7  "IdleSpeedIncrease_El"
  %iodicElLoad_B_Stat/1 -> bus_creator/8  "%iodicElLoad_B_Stat"
  PwSysULoFalt_D_Stat/1 -> bus_creator/9  "PwSysULoFalt_D_Stat"
  Shed_Drain_Eng_Off_B/1 -> bus_creator/10  "Shed_Drain_Eng_Off_B"
  Shed_Feature_Group_ID/1 -> bus_creator/11  "Shed_Feature_Group_ID"
  Shed_Level_Req/1 -> bus_creator/12  "Shed_Level_Req"
  Shed_T_Eng_Off_B/1 -> bus_creator/13  "Shed_T_Eng_Off_B"
  ULoRgenTestMde_B_Rq/1 -> bus_creator/14  "ULoRgenTestMde_B_Rq"

== system test_mdl1/VehicleCAN/GWM/Battery_Mgmt_3_FD1 ==
  BSBattQCapAh : Constant  Value=0
  BSBattQDeltaRideAh : Constant  Value=0
  BSBattSOC : Constant  Value=0
  BSFault : Constant  Value=0
  BattULo2_Te_Actl : Constant  Value=0
  BattULoChrg_URate_RqMx : Constant  Value=0
  BattULoChrg_U_RqMn : Constant  Value=0
  BattULoChrg_U_RqMx : Constant  Value=0
  BattULoState_D_Qlty : Constant  Value=0
  bus_creator : BusCreator  Inputs=9
  out_port : Outport
  wires:
  bus_creator/1 -> out_port/1  "test_mdl1"
  BSBattQCapAh/1 -> bus_creator/1  "BSBattQCapAh"
  BSBattQDeltaRideAh/1 -> bus_creator/2  "BSBattQDeltaRideAh"
  BSBattSOC/1 -> bus_creator/3  "BSBattSOC"
  BSFault/1 -> bus_creator/4  "BSFault"
  BattULo2_Te_Actl/1 -> bus_creator/5  "BattULo2_Te_Actl"
  BattULoChrg_URate_RqMx/1 -> bus_creator/6  "BattULoChrg_URate_RqMx"
  BattULoChrg_U_RqMn/1 -> bus_creator/7  "BattULoChrg_U_RqMn"
  BattULoChrg_U_RqMx/1 -> bus_creator/8  "BattULoChrg_U_RqMx"
  BattULoState_D_Qlty/1 -> bus_creator/9  "BattULoState_D_Qlty"

== system test_mdl1/VehicleCAN/GWM/Battery_Mgmt_4_FD1 ==
  BattULoAuxIsol_D_Rq : Constant  Value=0
  BattULoAuxSoc_Pc_Actl : Constant  Value=0
  BattULoAux_B_Falt : Constant  Value=0
  BattULoAux_D_Qlty : Constant  Value=0
  BattULoAux_I_Actl : Constant  Value=0
  BattULoAux_U_Actl : Constant  Value=0
  BattULoAux_U_Rq : Constant  Value=0
  BattULoCrnkBelt_U_Pred : Constant  Value=0
  BattULoCrnkStrt_U_Pred : Constant  Value=0
  bus_creator : BusCreator  Inputs=9
  out_port : Outport
  wires:
  bus_creator/1 -> out_port/1  "test_mdl1"
  BattULoAuxIsol_D_Rq/1 -> bus_creator/1  "BattULoAuxIsol_D_Rq"
  BattULoAuxSoc_Pc_Actl/1 -> bus_creator/2  "BattULoAuxSoc_Pc_Actl"
  BattULoAux_B_Falt/1 -> bus_creator/3  "BattULoAux_B_Falt"
  BattULoAux_D_Qlty/1 -> bus_creator/4  "BattULoAux_D_Qlty"
  BattULoAux_I_Actl/1 -> bus_creator/5  "BattULoAux_I_Actl"
  BattULoAux_U_Actl/1 -> bus_creator/6  "BattULoAux_U_Actl"
  BattULoAux_U_Rq/1 -> bus_creator/7  "BattULoAux_U_Rq"
  BattULoCrnkBelt_U_Pred/1 -> bus_creator/8  "BattULoCrnkBelt_U_Pred"
  BattULoCrnkStrt_U_Pred/1 -> bus_creator/9  "BattULoCrnkStrt_U_Pred"

== system test_mdl1/VehicleCAN/GWM/Battery_Traction_1_FD1 ==
  BattTracMil_D_Rq : Constant  Value=0
  BattTracOffFst_D_Actl : Constant  Value=0
  BattTracOff_B_Actl : Constant  Value=0
  BattTrac_I_Actl : Constant  Value=0
  BattTrac_U_Actl : Constant  Value=0
  BattTrac_U_LimHi : Constant  Value=0
  BattTrac_U_LimLo : Constant  Value=0
  VehStrtInhbt_B_RqBatt : Constant  Value=0
  bus_creator : BusCreator  Inputs=8
  out_port : Outport
  wires:
  bus_creator/1 -> out_port/1  "test_mdl1"
  BattTracMil_D_Rq/1 -> bus_creator/1  "BattTracMil_D_Rq"
  BattTracOffFst_D_Actl/1 -> bus_creator/2  "BattTracOffFst_D_Actl"
  BattTracOff_B_Actl/1 -> bus_creator/3  "BattTracOff_B_Actl"
  BattTrac_I_Actl/1 -> bus_creator/4  "BattTrac_I_Actl"
  BattTrac_U_Actl/1 -> bus_creator/5  "BattTrac_U_Actl"
  BattTrac_U_LimHi/1 -> bus_creator/6  "BattTrac_U_LimHi"
  BattTrac_U_LimLo/1 -> bus_creator/7  "BattTrac_U_LimLo"
  VehStrtInhbt_B_RqBatt/1 -> bus_creator/8  "VehStrtInhbt_B_RqBatt"

== system test_mdl1/VehicleCAN/GWM/Battery_Traction_3_FD1 ==
  BattTracClnt_Te_Actl : Constant  Value=0
  BattTracSoc_Pc_LimHi : Constant  Value=0
  BattTracSoc_Pc_LimLo : Constant  Value=0
  BattTracSoc_Pc_MnPrtct : Constant  Value=0
  BattTracSoc_Pc_MxPrtct : Constant  Value=0
  BattTracSrvcRqd_B_Rq : Constant  Value=0
  BattTracWarnLamp_B_Rq : Constant  Value=0
  bus_creator : BusCreator  Inputs=7
  out_port : Outport
  wires:
  bus_creator/1 -> out_port/1  "test_mdl1"
  BattTracClnt_Te_Actl/1 -> bus_creator/1  "BattTracClnt_Te_Actl"
  BattTracSoc_Pc_LimHi/1 -> bus_creator/2  "BattTracSoc_Pc_LimHi"
  BattTracSoc_Pc_LimLo/1 -> bus_creator/3  "BattTracSoc_Pc_LimLo"
  BattTracSoc_Pc_MnPrtct/1 -> bus_creator/4  "BattTracSoc_Pc_MnPrtct"
  BattTracSoc_Pc_MxPrtct/1 -> bus_creator/5  "BattTracSoc_Pc_MxPrtct"
  BattTracSrvcRqd_B_Rq/1 -> bus_creator/6  "BattTracSrvcRqd_B_Rq"
  BattTracWarnLamp_B_Rq/1 -> bus_creator/7  "BattTracWarnLamp_B_Rq"

== system test_mdl1/VehicleCAN/GWM/Battery_Traction_4_FD1 ==
  BattTracDiagClr_B_Rq : Constant  Value=0
  BattTracSoc2_Pc_Actl : Constant  Value=0
  BattTrac_Te_Actl : Constant  Value=0
  bus_creator : BusCreator  Inputs=3
  out_port : Outport
  wires:
  bus_creator/1 -> out_port/1  "test_mdl1"
  BattTracDiagClr_B_Rq/1 -> bus_creator/1  "BattTracDiagClr_B_Rq"
  BattTracSoc2_Pc_Actl/1 -> bus_creator/2  "BattTracSoc2_Pc_Actl"
  BattTrac_Te_Actl/1 -> bus_creator/3  "BattTrac_Te_Actl"

== system test_mdl1/VehicleCAN/GWM/Battery_Traction_5_FD1 ==
  BattTrac2_Pw_ChrgInst : Constant  Value=0
  BattTrac2_Pw_DchrgInst : Constant  Value=0
  BattTrac2_Pw_LimChrg : Constant  Value=0
  BattTrac2_Pw_LimDchrg : Constant  Value=0
  bus_creator : BusCreator  Inputs=4
  out_port : Outport
  wires:
  bus_creator/1 -> out_port/1  "test_mdl1"
  BattTrac2_Pw_ChrgInst/1 -> bus_creator/1  "BattTrac2_Pw_ChrgInst"
  BattTrac2_Pw_DchrgInst/1 -> bus_creator/2  "BattTrac2_Pw_DchrgInst"
  BattTrac2_Pw_LimChrg/1 -> bus_creator/3  "BattTrac2_Pw_LimChrg"
  BattTrac2_Pw_LimDchrg/1 -> bus_creator/4  "BattTrac2_Pw_LimDchrg"

== system test_mdl1/VehicleCAN/GWM/Battery_Traction_6_FD1 ==
  BattTracChrgSustn_B_Rq : Constant  Value=0
  BattTracClntPmp_D_Stat : Constant  Value=0
  BattTracCnnct_D_Cmd : Constant  Value=0
  BattTracDcdcDis_B_Rq : Constant  Value=0
  BattTracDelta_Te_Actl : Constant  Value=0
  BattTracHvilOpen_B_Stat : Constant  Value=0
  HtrnClntPump_D_Stat : Constant  Value=0
  bus_creator : BusCreator  Inputs=7
  out_port : Outport
  wires:
  bus_creator/1 -> out_port/1  "test_mdl1"
  BattTracChrgSustn_B_Rq/1 -> bus_creator/1  "BattTracChrgSustn_B_Rq"
  BattTracClntPmp_D_Stat/1 -> bus_creator/2  "BattTracClntPmp_D_Stat"
  BattTracCnnct_D_Cmd/1 -> bus_creator/3  "BattTracCnnct_D_Cmd"
  BattTracDcdcDis_B_Rq/1 -> bus_creator/4  "BattTracDcdcDis_B_Rq"
  BattTracDelta_Te_Actl/1 -> bus_creator/5  "BattTracDelta_Te_Actl"
  BattTracHvilOpen_B_Stat/1 -> bus_creator/6  "BattTracHvilOpen_B_Stat"
  HtrnClntPump_D_Stat/1 -> bus_creator/7  "HtrnClntPump_D_Stat"

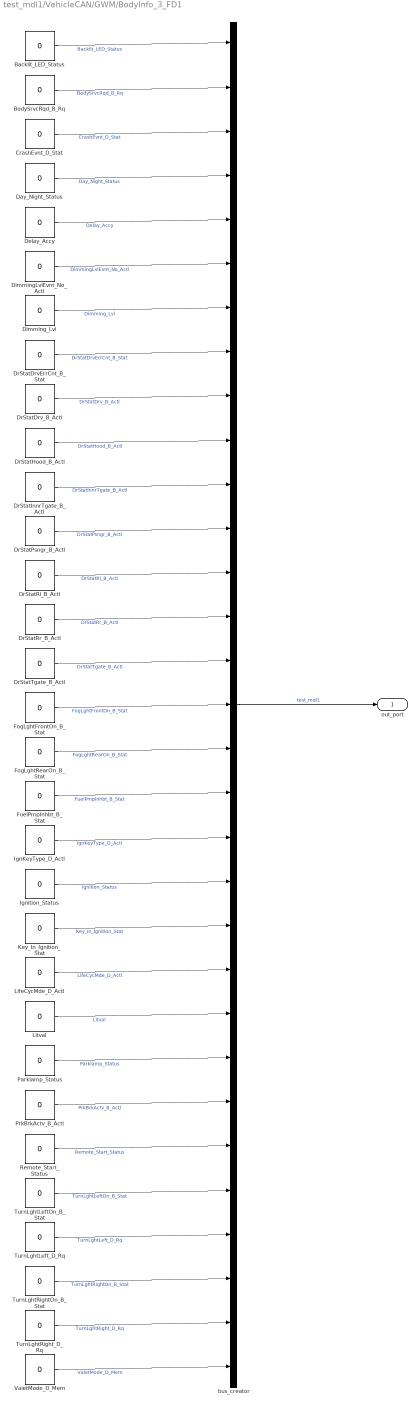
== system test_mdl1/VehicleCAN/GWM/BodyInfo_3_FD1 ==
  Backlit_LED_Status : Constant  Value=0
  BodySrvcRqd_B_Rq : Constant  Value=0
  CrashEvnt_D_Stat : Constant  Value=0
  Day_Night_Status : Constant  Value=0
  Delay_Accy : Constant  Value=0
  DimmingLvlEvnt_No_Actl : Constant  Value=0
  Dimming_Lvl : Constant  Value=0
  DrStatDrvErrCnt_B_Stat : Constant  Value=0
  DrStatDrv_B_Actl : Constant  Value=0
  DrStatHood_B_Actl : Constant  Value=0
  DrStatInnrTgate_B_Actl : Constant  Value=0
  DrStatPsngr_B_Actl : Constant  Value=0
  DrStatRl_B_Actl : Constant  Value=0
  DrStatRr_B_Actl : Constant  Value=0
  DrStatTgate_B_Actl : Constant  Value=0
  FogLghtFrontOn_B_Stat : Constant  Value=0
  FogLghtRearOn_B_Stat : Constant  Value=0
  FuelPmpInhbt_B_Stat : Constant  Value=0
  IgnKeyType_D_Actl : Constant  Value=0
  Ignition_Status : Constant  Value=0
  Key_In_Ignition_Stat : Constant  Value=0
  LifeCycMde_D_Actl : Constant  Value=0
  Litval : Constant  Value=0
  Parklamp_Status : Constant  Value=0
  PrkBrkActv_B_Actl : Constant  Value=0
  Remote_Start_Status : Constant  Value=0
  TurnLghtLeftOn_B_Stat : Constant  Value=0
  TurnLghtLeft_D_Rq : Constant  Value=0
  TurnLghtRightOn_B_Stat : Constant  Value=0
  TurnLghtRight_D_Rq : Constant  Value=0
  ValetMode_D_Mem : Constant  Value=0
  bus_creator : BusCreator  Inputs=31
  out_port : Outport
  wires:
  bus_creator/1 -> out_port/1  "test_mdl1"
  Backlit_LED_Status/1 -> bus_creator/1  "Backlit_LED_Status"
  BodySrvcRqd_B_Rq/1 -> bus_creator/2  "BodySrvcRqd_B_Rq"
  CrashEvnt_D_Stat/1 -> bus_creator/3  "CrashEvnt_D_Stat"
  Day_Night_Status/1 -> bus_creator/4  "Day_Night_Status"
  Delay_Accy/1 -> bus_creator/5  "Delay_Accy"
  DimmingLvlEvnt_No_Actl/1 -> bus_creator/6  "DimmingLvlEvnt_No_Actl"
  Dimming_Lvl/1 -> bus_creator/7  "Dimming_Lvl"
  DrStatDrvErrCnt_B_Stat/1 -> bus_creator/8  "DrStatDrvErrCnt_B_Stat"
  DrStatDrv_B_Actl/1 -> bus_creator/9  "DrStatDrv_B_Actl"
  DrStatHood_B_Actl/1 -> bus_creator/10  "DrStatHood_B_Actl"
  DrStatInnrTgate_B_Actl/1 -> bus_creator/11  "DrStatInnrTgate_B_Actl"
  DrStatPsngr_B_Actl/1 -> bus_creator/12  "DrStatPsngr_B_Actl"
  DrStatRl_B_Actl/1 -> bus_creator/13  "DrStatRl_B_Actl"
  DrStatRr_B_Actl/1 -> bus_creator/14  "DrStatRr_B_Actl"
  DrStatTgate_B_Actl/1 -> bus_creator/15  "DrStatTgate_B_Actl"
  FogLghtFrontOn_B_Stat/1 -> bus_creator/16  "FogLghtFrontOn_B_Stat"
  FogLghtRearOn_B_Stat/1 -> bus_creator/17  "FogLghtRearOn_B_Stat"
  FuelPmpInhbt_B_Stat/1 -> bus_creator/18  "FuelPmpInhbt_B_Stat"
  IgnKeyType_D_Actl/1 -> bus_creator/19  "IgnKeyType_D_Actl"
  Ignition_Status/1 -> bus_creator/20  "Ignition_Status"
  Key_In_Ignition_Stat/1 -> bus_creator/21  "Key_In_Ignition_Stat"
  LifeCycMde_D_Actl/1 -> bus_creator/22  "LifeCycMde_D_Actl"
  Litval/1 -> bus_creator/23  "Litval"
  Parklamp_Status/1 -> bus_creator/24  "Parklamp_Status"
  PrkBrkActv_B_Actl/1 -> bus_creator/25  "PrkBrkActv_B_Actl"
  Remote_Start_Status/1 -> bus_creator/26  "Remote_Start_Status"
  TurnLghtLeftOn_B_Stat/1 -> bus_creator/27  "TurnLghtLeftOn_B_Stat"
  TurnLghtLeft_D_Rq/1 -> bus_creator/28  "TurnLghtLeft_D_Rq"
  TurnLghtRightOn_B_Stat/1 -> bus_creator/29  "TurnLghtRightOn_B_Stat"
  TurnLghtRight_D_Rq/1 -> bus_creator/30  "TurnLghtRight_D_Rq"
  ValetMode_D_Mem/1 -> bus_creator/31  "ValetMode_D_Mem"

== system test_mdl1/VehicleCAN/GWM/Body_Info_10_FD1 ==
  GenericSwtch1_No_Actl : Constant  Value=0
  GenericSwtch2_No_Actl : Constant  Value=0
  GenericSwtch3_No_Actl : Constant  Value=0
  bus_creator : BusCreator  Inputs=3
  out_port : Outport
  wires:
  bus_creator/1 -> out_port/1  "test_mdl1"
  GenericSwtch1_No_Actl/1 -> bus_creator/1  "GenericSwtch1_No_Actl"
  GenericSwtch2_No_Actl/1 -> bus_creator/2  "GenericSwtch2_No_Actl"
  GenericSwtch3_No_Actl/1 -> bus_creator/3  "GenericSwtch3_No_Actl"

== system test_mdl1/VehicleCAN/GWM/Body_Info_4_FD1 ==
  BattULo_I_Actl : Constant  Value=0
  BattULo_U_Actl : Constant  Value=0
  BrkTrnShifLck_B_Stat : Constant  Value=0
  DcacElPw_D_Rq : Constant  Value=0
  DriverCrankingReq : Constant  Value=0
  EngOff_T_Actl : Constant  Value=0
  FuelPumpPwr_D_Stat : Constant  Value=0
  PrkLckCtlAvail_T_Stat : Constant  Value=0
  PrkLckCtlMsgTxt_D_Rq : Constant  Value=0
  PrkLckCtlTow_B_Enbl : Constant  Value=0
  PrkLckCtlUnlck_D_Stat : Constant  Value=0
  PrkLckCtl_B_Enbl : Constant  Value=0
  PtLatchActv_B_RqBcm : Constant  Value=0
  ReFuelSwtchStat_D_Actl : Constant  Value=0
  bus_creator : BusCreator  Inputs=15
  immoSecureIdleMode : Constant  Value=0
  out_port : Outport
  wires:
  bus_creator/1 -> out_port/1  "test_mdl1"
  BattULo_I_Actl/1 -> bus_creator/1  "BattULo_I_Actl"
  BattULo_U_Actl/1 -> bus_creator/2  "BattULo_U_Actl"
  BrkTrnShifLck_B_Stat/1 -> bus_creator/3  "BrkTrnShifLck_B_Stat"
  DcacElPw_D_Rq/1 -> bus_creator/4  "DcacElPw_D_Rq"
  DriverCrankingReq/1 -> bus_creator/5  "DriverCrankingReq"
  EngOff_T_Actl/1 -> bus_creator/6  "EngOff_T_Actl"
  FuelPumpPwr_D_Stat/1 -> bus_creator/7  "FuelPumpPwr_D_Stat"
  PrkLckCtlAvail_T_Stat/1 -> bus_creator/8  "PrkLckCtlAvail_T_Stat"
  PrkLckCtlMsgTxt_D_Rq/1 -> bus_creator/9  "PrkLckCtlMsgTxt_D_Rq"
  PrkLckCtlTow_B_Enbl/1 -> bus_creator/10  "PrkLckCtlTow_B_Enbl"
  PrkLckCtlUnlck_D_Stat/1 -> bus_creator/11  "PrkLckCtlUnlck_D_Stat"
  PrkLckCtl_B_Enbl/1 -> bus_creator/12  "PrkLckCtl_B_Enbl"
  PtLatchActv_B_RqBcm/1 -> bus_creator/13  "PtLatchActv_B_RqBcm"
  ReFuelSwtchStat_D_Actl/1 -> bus_creator/14  "ReFuelSwtchStat_D_Actl"
  immoSecureIdleMode/1 -> bus_creator/15  "immoSecureIdleMode"

== system test_mdl1/VehicleCAN/GWM/Body_Info_6_FD1 ==
  DrLatchMsgTxt_D_Rq : Constant  Value=0
  ElPwPoint_D_Rq : Constant  Value=0
  HeadLghtHiPrmsn_D_Stat : Constant  Value=0
  IgnPsswrdDsply_B_Rq : Constant  Value=0
  KeyAdmnTot_No_Cnt : Constant  Value=0
  KeyMykeyTot_No_Cnt : Constant  Value=0
  Keycode_Status : Constant  Value=0
  PEBackupSlot_Stats : Constant  Value=0
  PoliceIdlMde_D_Stat : Constant  Value=0
  PrmtrAlrmEvnt_D_Stat : Constant  Value=0
  PrsnlDevcChrgEnbl_B_Rq : Constant  Value=0
  SecurityMsgTxt_D_Rq : Constant  Value=0
  SteWhlLckMsgTxt_D_Rq : Constant  Value=0
  TracKeyMde_D_Stat : Constant  Value=0
  bus_creator : BusCreator  Inputs=15
  immoMsgTxt_D_Rq : Constant  Value=0
  out_port : Outport
  wires:
  bus_creator/1 -> out_port/1  "test_mdl1"
  DrLatchMsgTxt_D_Rq/1 -> bus_creator/1  "DrLatchMsgTxt_D_Rq"
  ElPwPoint_D_Rq/1 -> bus_creator/2  "ElPwPoint_D_Rq"
  HeadLghtHiPrmsn_D_Stat/1 -> bus_creator/3  "HeadLghtHiPrmsn_D_Stat"
  IgnPsswrdDsply_B_Rq/1 -> bus_creator/4  "IgnPsswrdDsply_B_Rq"
  KeyAdmnTot_No_Cnt/1 -> bus_creator/5  "KeyAdmnTot_No_Cnt"
  KeyMykeyTot_No_Cnt/1 -> bus_creator/6  "KeyMykeyTot_No_Cnt"
  Keycode_Status/1 -> bus_creator/7  "Keycode_Status"
  PEBackupSlot_Stats/1 -> bus_creator/8  "PEBackupSlot_Stats"
  PoliceIdlMde_D_Stat/1 -> bus_creator/9  "PoliceIdlMde_D_Stat"
  PrmtrAlrmEvnt_D_Stat/1 -> bus_creator/10  "PrmtrAlrmEvnt_D_Stat"
  PrsnlDevcChrgEnbl_B_Rq/1 -> bus_creator/11  "PrsnlDevcChrgEnbl_B_Rq"
  SecurityMsgTxt_D_Rq/1 -> bus_creator/12  "SecurityMsgTxt_D_Rq"
  SteWhlLckMsgTxt_D_Rq/1 -> bus_creator/13  "SteWhlLckMsgTxt_D_Rq"
  TracKeyMde_D_Stat/1 -> bus_creator/14  "TracKeyMde_D_Stat"
  immoMsgTxt_D_Rq/1 -> bus_creator/15  "immoMsgTxt_D_Rq"

== system test_mdl1/VehicleCAN/GWM/Body_Info_8_FD1 ==
  BattRgenLoChrg_D_Rq : Constant  Value=0
  BattRgenLoDChrg_D_Rq : Constant  Value=0
  ChrgCordLck_B_Stat : Constant  Value=0
  ChrgCordResp1_No_Actl : Constant  Value=0
  ChrgCordResp2_No_Actl : Constant  Value=0
  WakeAlarm0_D_Stat : Constant  Value=0
  WakeAlarm1_D_Stat : Constant  Value=0
  WakeAlarm2_D_Stat : Constant  Value=0
  WakeAlarm3_D_Stat : Constant  Value=0
  bus_creator : BusCreator  Inputs=9
  out_port : Outport
  wires:
  bus_creator/1 -> out_port/1  "test_mdl1"
  BattRgenLoChrg_D_Rq/1 -> bus_creator/1  "BattRgenLoChrg_D_Rq"
  BattRgenLoDChrg_D_Rq/1 -> bus_creator/2  "BattRgenLoDChrg_D_Rq"
  ChrgCordLck_B_Stat/1 -> bus_creator/3  "ChrgCordLck_B_Stat"
  ChrgCordResp1_No_Actl/1 -> bus_creator/4  "ChrgCordResp1_No_Actl"
  ChrgCordResp2_No_Actl/1 -> bus_creator/5  "ChrgCordResp2_No_Actl"
  WakeAlarm0_D_Stat/1 -> bus_creator/6  "WakeAlarm0_D_Stat"
  WakeAlarm1_D_Stat/1 -> bus_creator/7  "WakeAlarm1_D_Stat"
  WakeAlarm2_D_Stat/1 -> bus_creator/8  "WakeAlarm2_D_Stat"
  WakeAlarm3_D_Stat/1 -> bus_creator/9  "WakeAlarm3_D_Stat"

== system test_mdl1/VehicleCAN/GWM/Body_Info_9_FD1 ==
  AdvStrt_D_Stat : Constant  Value=0
  CrnkInhbt_B_Stat : Constant  Value=0
  CrnkInhbt_No_Cnt : Constant  Value=0
  CrnkInhbt_No_Cs : Constant  Value=0
  DrvInCtl_B_Stat : Constant  Value=0
  EngStrtActv_B_Stat : Constant  Value=0
  EngStrt_B_Rq : Constant  Value=0
  IgnPreOffActv_B_Stat : Constant  Value=0
  PtWakeReas_D_Stat : Constant  Value=0
  StrtrMtrCtlDStat_No_Cs : Constant  Value=0
  VehOnSrc_D_Stat : Constant  Value=0
  bus_creator : BusCreator  Inputs=11
  out_port : Outport
  wires:
  bus_creator/1 -> out_port/1  "test_mdl1"
  AdvStrt_D_Stat/1 -> bus_creator/1  "AdvStrt_D_Stat"
  CrnkInhbt_B_Stat/1 -> bus_creator/2  "CrnkInhbt_B_Stat"
  CrnkInhbt_No_Cnt/1 -> bus_creator/3  "CrnkInhbt_No_Cnt"
  CrnkInhbt_No_Cs/1 -> bus_creator/4  "CrnkInhbt_No_Cs"
  DrvInCtl_B_Stat/1 -> bus_creator/5  "DrvInCtl_B_Stat"
  EngStrtActv_B_Stat/1 -> bus_creator/6  "EngStrtActv_B_Stat"
  EngStrt_B_Rq/1 -> bus_creator/7  "EngStrt_B_Rq"
  IgnPreOffActv_B_Stat/1 -> bus_creator/8  "IgnPreOffActv_B_Stat"
  PtWakeReas_D_Stat/1 -> bus_creator/9  "PtWakeReas_D_Stat"
  StrtrMtrCtlDStat_No_Cs/1 -> bus_creator/10  "StrtrMtrCtlDStat_No_Cs"
  VehOnSrc_D_Stat/1 -> bus_creator/11  "VehOnSrc_D_Stat"
